simulink library "LibExpRefLookup"  (R2019b)
settings: Solver=VariableStepAuto  StartTime=0.0  StopTime=10.0  RelTol=1e-3
undefined symbols (not defined in the file or in its folder): refAccelPedalCmd, refAccelPedalDBW, refAxleTorq, refBattCurr, refBattSoc, refBattVolt, refBrakePedalCmd, refBrakePredalDBW, refSpare1, refSpare2, refSpare3, refSpare4, refSpare5, refSpare6, refTime, refVehSpd
settings Model: Creator=y0n  LastModifiedBy=y0n

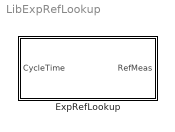
== system LibExpRefLookup ==
  ExpRefLookup : Subsystem

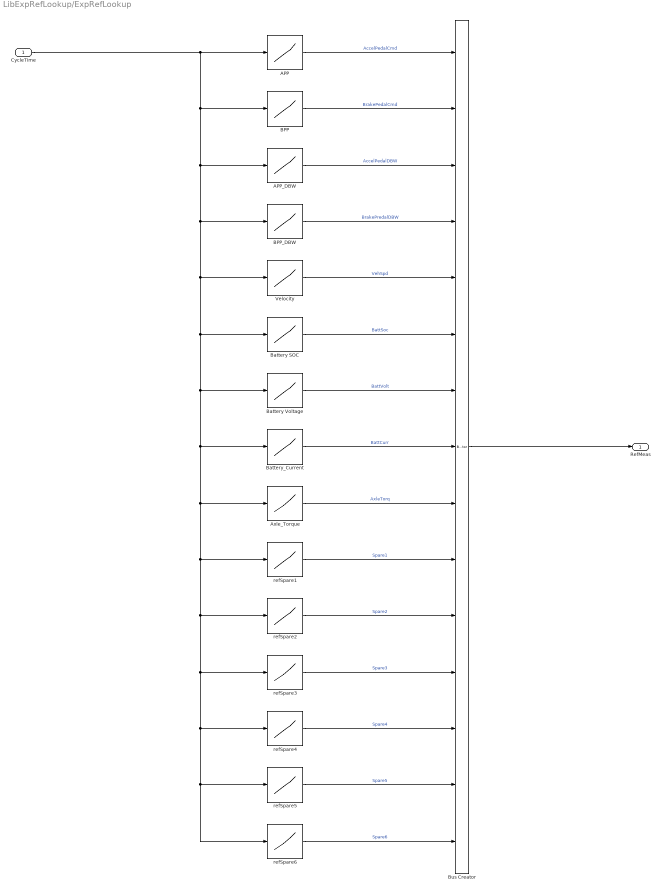
== system LibExpRefLookup/ExpRefLookup ==
  CycleTime : Inport
  APP : Lookup_n-D  NumberOfTableDimensions=1  BreakpointsForDimension1=refTime  Table=refAccelPedalCmd  InternalRulePriority=Speed  RndMeth=Simplest  InputSameDT=on
  APP_DBW : Lookup_n-D  NumberOfTableDimensions=1  BreakpointsForDimension1=refTime  Table=refAccelPedalDBW  InternalRulePriority=Speed  RndMeth=Simplest  InputSameDT=on
  Axle_Torque : Lookup_n-D  NumberOfTableDimensions=1  BreakpointsForDimension1=refTime  Table=refAxleTorq  InternalRulePriority=Speed  RndMeth=Simplest  InputSameDT=on
  BPP : Lookup_n-D  NumberOfTableDimensions=1  BreakpointsForDimension1=refTime  Table=refBrakePedalCmd  InternalRulePriority=Speed  RndMeth=Simplest  InputSameDT=on
  BPP_DBW : Lookup_n-D  NumberOfTableDimensions=1  BreakpointsForDimension1=refTime  Table=refBrakePredalDBW  InternalRulePriority=Speed  RndMeth=Simplest  InputSameDT=on
  Battery SOC : Lookup_n-D  NumberOfTableDimensions=1  BreakpointsForDimension1=refTime  Table=refBattSoc  InternalRulePriority=Speed  RndMeth=Simplest  InputSameDT=on
  Battery Voltage : Lookup_n-D  NumberOfTableDimensions=1  BreakpointsForDimension1=refTime  Table=refBattVolt  InternalRulePriority=Speed  RndMeth=Simplest  InputSameDT=on
  Battery_Current : Lookup_n-D  NumberOfTableDimensions=1  BreakpointsForDimension1=refTime  Table=refBattCurr  InternalRulePriority=Speed  RndMeth=Simplest  InputSameDT=on
  Bus Creator : BusCreator  Inputs=15
  Velocity : Lookup_n-D  NumberOfTableDimensions=1  BreakpointsForDimension1=refTime  Table=refVehSpd  InternalRulePriority=Speed  RndMeth=Simplest  InputSameDT=on
  refSpare1 : Lookup_n-D  NumberOfTableDimensions=1  BreakpointsForDimension1=refTime  Table=refSpare1  InternalRulePriority=Speed  RndMeth=Simplest  InputSameDT=on
  refSpare2 : Lookup_n-D  NumberOfTableDimensions=1  BreakpointsForDimension1=refTime  Table=refSpare2  InternalRulePriority=Speed  RndMeth=Simplest  InputSameDT=on
  refSpare3 : Lookup_n-D  NumberOfTableDimensions=1  BreakpointsForDimension1=refTime  Table=refSpare3  InternalRulePriority=Speed  RndMeth=Simplest  InputSameDT=on
  refSpare4 : Lookup_n-D  NumberOfTableDimensions=1  BreakpointsForDimension1=refTime  Table=refSpare4  InternalRulePriority=Speed  RndMeth=Simplest  InputSameDT=on
  refSpare5 : Lookup_n-D  NumberOfTableDimensions=1  BreakpointsForDimension1=refTime  Table=refSpare5  InternalRulePriority=Speed  RndMeth=Simplest  InputSameDT=on
  refSpare6 : Lookup_n-D  NumberOfTableDimensions=1  BreakpointsForDimension1=refTime  Table=refSpare6  InternalRulePriority=Speed  RndMeth=Simplest  InputSameDT=on
  RefMeas : Outport
  wires:
  CycleTime/1 -> refSpare4/1, refSpare5/1, refSpare6/1, refSpare3/1, refSpare2/1, refSpare1/1, Axle_Torque/1, Battery_Current/1, Battery Voltage/1, Battery SOC/1, Velocity/1, BPP_DBW/1, APP_DBW/1, BPP/1, APP/1
  refSpare3/1 -> Bus Creator/12  "Spare3"
  Velocity/1 -> Bus Creator/5  "VehSpd"
  Battery Voltage/1 -> Bus Creator/7  "BattVolt"
  Axle_Torque/1 -> Bus Creator/9  "AxleTorq"
  refSpare6/1 -> Bus Creator/15  "Spare6"
  APP/1 -> Bus Creator/1  "AccelPedalCmd"
  refSpare1/1 -> Bus Creator/10  "Spare1"
  Battery SOC/1 -> Bus Creator/6  "BattSoc"
  refSpare2/1 -> Bus Creator/11  "Spare2"
  refSpare5/1 -> Bus Creator/14  "Spare5"
  BPP_DBW/1 -> Bus Creator/4  "BrakePredalDBW"
  Battery_Current/1 -> Bus Creator/8  "BattCurr"
  refSpare4/1 -> Bus Creator/13  "Spare4"
  APP_DBW/1 -> Bus Creator/3  "AccelPedalDBW"
  BPP/1 -> Bus Creator/2  "BrakePedalCmd"
  Bus Creator/1 -> RefMeas/1
